simulink model "Route_Generator"  (R2016b)
settings: Solver=FixedStepDiscrete  StartTime=0.0  StopTime=inf  FixedStep=RouteGenr.tiSimnTiStep_C  RelTol=1e-3  EnableMultiTasking=on
undefined symbols (not defined in the file or in its folder): gui_data
settings Model: Creator=sevren  LastModifiedBy=sevren
settings DataIOCC: SaveFormat=StructureWithTime  SaveOutput=off  DSMLogging=off  VisualizeSimOutput=off  SaveTime=off  SignalLoggingName=Results
settings OptimizationCC: BlockReduction=off  ConditionallyExecuteInputs=off  LifeSpan=inf
settings DebuggingCC: AllowSymbolicDim=off  SFUnexpectedBacktrackingDiag=warning  SFNoUnconditionalDefaultTransitionDiag=warning  SFExecutionAtInitializationDiag=none
settings ModelReferenceCC: ModelReferenceNumInstancesAllowed=Single  PropagateSignalLabelsOutOfModel=off
settings GRTTargetCC: TargetLangStandard=C89/C90 (ANSI)
settings ConfigComp: CovMetricSettings=dw  CovHtmlReporting=on  CovSaveCumulativeToWorkspaceVar=on  CovSaveSingleToWorkspaceVar=on  CovExternalEMLEnable=off

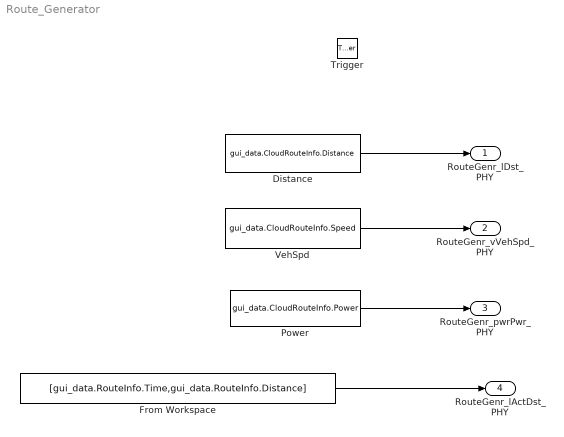
== system Route_Generator ==
  Trigger : TriggerPort  TriggerType=function-call  VariantControl=Variant  PortDimensions=1
  Distance : Constant  Value=gui_data.CloudRouteInfo.Distance  SampleTime=-1
  From Workspace : FromWorkspace  VariableName=[gui_data.RouteInfo.Time,gui_data.RouteInfo.Distance]
  Power : Constant  Value=gui_data.CloudRouteInfo.Power  SampleTime=-1
  VehSpd : Constant  Value=gui_data.CloudRouteInfo.Speed  SampleTime=-1
  RouteGenr_lDst_PHY : Outport
  RouteGenr_vVehSpd_PHY : Outport  Port=2
  RouteGenr_pwrPwr_PHY : Outport  Port=3
  RouteGenr_lActDst_PHY : Outport  Port=4
  wires:
  Power/1 -> RouteGenr_pwrPwr_PHY/1
  VehSpd/1 -> RouteGenr_vVehSpd_PHY/1
  Distance/1 -> RouteGenr_lDst_PHY/1
  From Workspace/1 -> RouteGenr_lActDst_PHY/1
